simulink model "rosen"  (R2013a)
settings: Solver=ode45  StartTime=0.0  StopTime=10.0  RelTol=1e-3
settings Model: Creator=haresh  LastModifiedBy=haresh

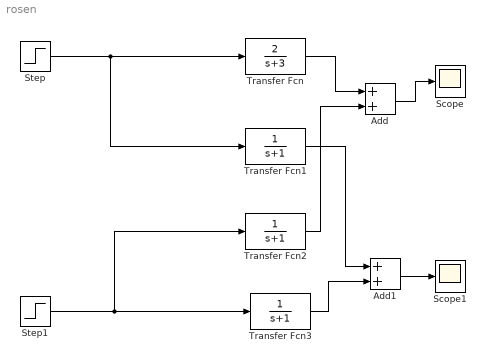
== system rosen ==
  Add : Sum
  Add1 : Sum
  Scope : Scope
  Scope1 : Scope
  Step : Step  Time=0  After=5  SampleTime=0
  Step1 : Step  Time=0  After=5  SampleTime=0
  Transfer Fcn : TransferFcn  Numerator=[2]  Denominator=[1 3]
  Transfer Fcn1 : TransferFcn  Denominator=[1 1]
  Transfer Fcn2 : TransferFcn  Denominator=[1 1]
  Transfer Fcn3 : TransferFcn  Denominator=[1 1]
  wires:
  Step/1 -> Transfer Fcn1/1, Transfer Fcn/1
  Step1/1 -> Transfer Fcn2/1, Transfer Fcn3/1
  Transfer Fcn/1 -> Add/1
  Transfer Fcn2/1 -> Add/2
  Transfer Fcn1/1 -> Add1/1
  Transfer Fcn3/1 -> Add1/2
  Add/1 -> Scope/1
  Add1/1 -> Scope1/1
